simulink model "sampleModel1439"  (R2023a)
settings: Solver=VariableStepAuto  StartTime=0.0  StopTime=10.0  RelTol=1e-3
libraries: hdlsllib x4, simulink x1
settings Model: Creator=user1  LastModifiedBy=user1

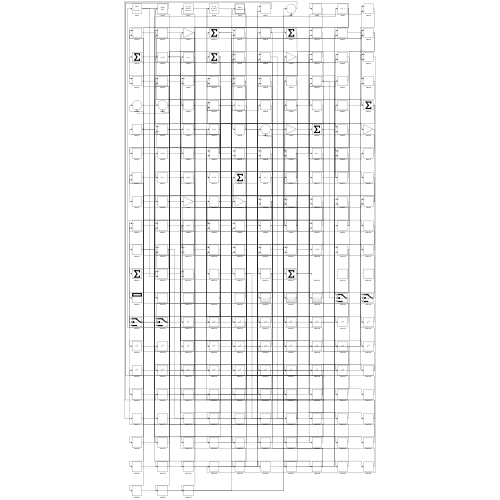
[thumbnail: Simulink's stored preview of the top-level diagram]
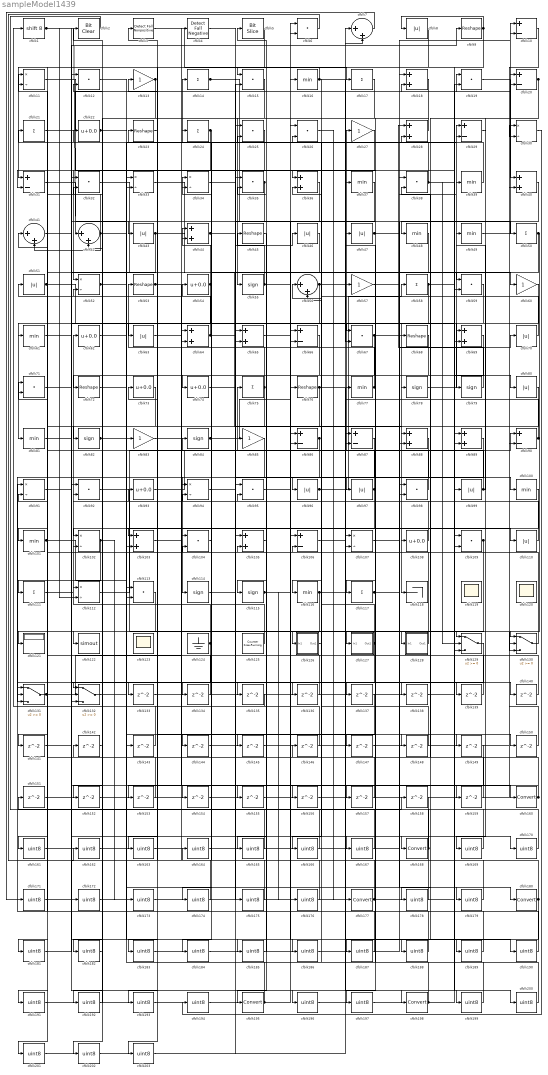
== system sampleModel1439 ==
  cfblk1 : ArithShift  BitShiftNumber=8
  cfblk{10,20,29,31,66,86..87,90,106} (9 alike) : Sum  Inputs=+-
  cfblk{16,37,39,48..49,61,77,81,100..101,116} (11 alike) : MinMax
  cfblk{11,30,33..34,52,91,94,102,107,112} (10 alike) : Product  Inputs=*/  RndMeth=Zero  SaturateOnIntegerOverflow=on
  cfblk{18,28,36,40,44,64..65,69,88..89,103,105} (12 alike) : Sum
  cfblk{6,12,15,19,25..26,32,35,38,59,67,71,92,95,98,104,109,113} (18 alike) : DotProduct  OutDataTypeStr=Inherit: Inherit via internal rule
  cfblk{22,54,62,73..74,93,108} (7 alike) : Bias  Bias=0.0  SaturateOnIntegerOverflow=off
  cfblk{8,43,46..47,51,63,70,80,96..97,99,110} (12 alike) : Abs  SaturateOnIntegerOverflow=off
  cfblk{14,17,21,24,50,58,75,111,117} (9 alike) : Sum  Inputs=+
  cfblk{55,78..79,82,84,114..115} (7 alike) : Signum
  cfblk118 : Terminator
  cfblk119 : Scope
      settings: Floating=on
  cfblk120 : Scope
      settings: Floating=on
  cfblk121 : Display
  cfblk122 : ToWorkspace  VariableName=simout  SaveFormat=Timeseries  SampleTime=-1
  cfblk123 : Scope
      settings: Floating=on
  cfblk124 : Ground
  cfblk125 : hdlsllib/Sources/Counter Free-Running  NumBits=16  tsamp=-1
  cfblk126 : Subsystem
      settings: LibrarySourceBlock=|
      | hdlsllib/Ports &
      | Subsystems/Subsystem
  cfblk127 : Subsystem
      settings: LibrarySourceBlock=|
      | hdlsllib/Ports &
      | Subsystems/Subsystem
  cfblk128 : Subsystem
      settings: LibrarySourceBlock=|
      | hdlsllib/Ports &
      | Subsystems/Subsystem
  cfblk{129..132} (4 alike) : Switch  SaturateOnIntegerOverflow=off  InputSameDT=off
  cfblk{13,27,57,60,83,85} (6 alike) : Gain
  cfblk{133..159} (27 alike) : Delay  SampleTime=1
  cfblk{160,168,177,180,195,198} (6 alike) : DataTypeConversion  SaturateOnIntegerOverflow=off  RndMeth=Floor
  cfblk{161..167,169..176,178..179,181..194,196..197,199..203} (38 alike) : DataTypeConversion  OutDataTypeStr=uint8  SaturateOnIntegerOverflow=off  RndMeth=Floor
  cfblk2 : simulink/Logic and Bit Operations/Bit Clear  iBit=0
      settings: LibrarySourceBlock=|
      | hdlsllib/Logic and Bit
      | Operations/Bit Clear
  cfblk{9,23,45,53,68,72,76} (7 alike) : Reshape
  cfblk3 : hdlsllib/Logic and Bit Operations/Detect Fall Nonpositive  vinit=0  OutDataTypeStr=boolean
  cfblk4 : hdlsllib/Logic and Bit Operations/Detect Fall Negative  vinit=0  OutDataTypeStr=boolean
  cfblk{7,41..42,56} (4 alike) : Sum  Inputs=|++
  cfblk5 : hdlsllib/Logic and Bit Operations/Bit Slice  lidx=7  ridx=0
  wires:
  cfblk17/1 -> cfblk55/1
  cfblk40/1 -> cfblk48/1
  cfblk86/1 -> cfblk114/1, cfblk131/3
  cfblk54/1 -> cfblk81/1, cfblk44/2
  cfblk79/1 -> cfblk28/1
  cfblk28/1 -> cfblk36/1
  cfblk32/1 -> cfblk118/1
  cfblk24/1 -> cfblk52/1, cfblk184/1
  cfblk1/1 -> cfblk42/1, cfblk59/1, cfblk112/2
  cfblk49/1 -> cfblk10/1
  cfblk124/1 -> cfblk62/1, cfblk203/1
  cfblk75/1 -> cfblk53/1, cfblk101/1
  cfblk35/1 -> cfblk132/3, cfblk144/1
  cfblk52/1 -> cfblk33/2, cfblk157/1
  cfblk97/1 -> cfblk3/1, cfblk41/1, cfblk156/1
  cfblk31/1 -> cfblk83/1
  cfblk50/1 -> cfblk130/1, cfblk135/1
  cfblk55/1 -> cfblk45/1, cfblk69/2, cfblk130/3
  cfblk89/1 -> cfblk195/1
  cfblk51/1 -> cfblk108/1, cfblk185/1
  cfblk96/1 -> cfblk58/1, cfblk166/1
  cfblk5/1 -> cfblk31/1
  cfblk69/1 -> cfblk78/1
  cfblk58/1 -> cfblk61/1, cfblk150/1
  cfblk90/1 -> cfblk27/1, cfblk82/1
  cfblk116/1 -> cfblk149/1, cfblk161/1
  cfblk42/1 -> cfblk11/1, cfblk41/2, cfblk29/2
  cfblk38/1 -> cfblk14/1, cfblk80/1, cfblk129/2
  cfblk3/1 -> cfblk17/1
  cfblk98/1 -> cfblk37/1
  cfblk78/1 -> cfblk29/1
  cfblk110/1 -> cfblk2/1
  cfblk14/1 -> cfblk68/1, cfblk167/1
  cfblk43/1 -> cfblk121/1, cfblk67/2
  cfblk113/1 -> cfblk122/1
  cfblk44/1 -> cfblk88/1, cfblk107/2
  cfblk125/1 -> cfblk84/1
  cfblk101/1 -> cfblk143/1, cfblk170/1
  cfblk70/1 -> cfblk21/1
  cfblk93/1 -> cfblk75/1
  cfblk27/1 -> cfblk31/2
  cfblk128/1(Out1) -> cfblk73/1
  cfblk41/1 -> cfblk67/1
  cfblk47/1 -> cfblk97/1, cfblk10/2
  cfblk112/1 -> cfblk64/1
  cfblk15/1 -> cfblk72/1
  cfblk77/1 -> cfblk54/1, cfblk34/1
  cfblk59/1 -> cfblk116/1
  cfblk16/1 -> cfblk15/1, cfblk60/1, cfblk126/1(In1)
  cfblk115/1 -> cfblk19/1, cfblk176/1
  cfblk111/1 -> cfblk112/1
  cfblk23/1 -> cfblk63/1
  cfblk107/1 -> cfblk39/1
  cfblk102/1 -> cfblk111/1, cfblk173/1
  cfblk22/1 -> cfblk59/2, cfblk148/1
  cfblk19/1 -> cfblk40/1
  cfblk11/1 -> cfblk109/1
  cfblk56/1 -> cfblk28/2, cfblk133/1
  cfblk33/1 -> cfblk76/1
  cfblk72/1 -> cfblk110/1
  cfblk127/1(Out1) -> cfblk56/1, cfblk131/2
  cfblk60/1 -> cfblk79/1
  cfblk106/1 -> cfblk198/1
  cfblk18/1 -> cfblk117/1
  cfblk48/1 -> cfblk94/1
  cfblk109/1 -> cfblk129/1, cfblk163/1
  cfblk92/1 -> cfblk127/1(In1)
  cfblk53/1 -> cfblk139/1, cfblk140/1
  cfblk76/1 -> cfblk115/1, cfblk128/1(In1)
  cfblk57/1 -> cfblk160/1
  cfblk130/1 -> cfblk71/1
  cfblk103/1 -> cfblk90/1
  cfblk108/1 -> cfblk24/1
  cfblk84/1 -> cfblk16/1, cfblk34/2
  cfblk94/1 -> cfblk18/2
  cfblk67/1 -> cfblk74/1, cfblk20/2, cfblk103/2
  cfblk36/1 -> cfblk86/2
  cfblk82/1 -> cfblk132/1, cfblk147/1
  cfblk21/1 -> cfblk20/1
  cfblk71/1 -> cfblk9/1
  cfblk39/1 -> cfblk5/1
  cfblk95/1 -> cfblk168/1
  cfblk117/1 -> cfblk70/1, cfblk179/1
  cfblk20/1 -> cfblk69/1, cfblk188/1
  cfblk37/1 -> cfblk102/1
  cfblk13/1 -> cfblk113/2, cfblk202/1
  cfblk26/1 -> cfblk177/1
  cfblk10/1 -> cfblk30/2
  cfblk114/1 -> cfblk46/1
  cfblk64/1 -> cfblk51/1, cfblk88/2, cfblk13/1
  cfblk74/1 -> cfblk100/1
  cfblk131/1 -> cfblk4/1, cfblk154/1
  cfblk4/1 -> cfblk50/1
  cfblk9/1 -> cfblk43/1, cfblk103/1, cfblk8/1, cfblk129/3
  cfblk12/1 -> cfblk180/1
  cfblk99/1 -> cfblk49/1, cfblk44/1
  cfblk126/1(Out1) -> cfblk56/2
  cfblk68/1 -> cfblk96/1
  cfblk133/1 -> cfblk109/2
  cfblk46/1 -> cfblk134/1
  cfblk134/1 -> cfblk33/1
  cfblk135/1 -> cfblk1/1
  cfblk81/1 -> cfblk136/1
  cfblk136/1 -> cfblk92/1
  cfblk88/1 -> cfblk137/1
  cfblk83/1 -> cfblk138/1
  cfblk139/1 -> cfblk18/1
  cfblk140/1 -> cfblk11/2
  cfblk85/1 -> cfblk141/1
  cfblk142/1 -> cfblk52/2
  cfblk143/1 -> cfblk102/2
  cfblk144/1 -> cfblk86/1
  cfblk132/1 -> cfblk145/1
  cfblk145/1 -> cfblk30/1
  cfblk146/1 -> cfblk131/1
  cfblk147/1 -> cfblk90/2
  cfblk148/1 -> cfblk36/2
  cfblk150/1 -> cfblk130/2
  cfblk151/1 -> cfblk98/1
  cfblk80/1 -> cfblk152/1
  cfblk152/1 -> cfblk64/2
  cfblk153/1 -> cfblk71/2
  cfblk154/1 -> cfblk94/2
  cfblk45/1 -> cfblk155/1
  cfblk155/1 -> cfblk40/2
  cfblk156/1 -> cfblk19/2
  cfblk157/1 -> cfblk42/2
  cfblk2/1 -> cfblk158/1
  cfblk63/1 -> cfblk159/1
  cfblk159/1 -> cfblk23/1
  cfblk160/1 -> cfblk153/1, cfblk38/2
  cfblk161/1 -> cfblk57/1
  cfblk6/1 -> cfblk162/1
  cfblk162/1 -> cfblk98/2
  cfblk163/1 -> cfblk6/1
  cfblk158/1 -> cfblk164/1
  cfblk164/1 -> cfblk6/2
  cfblk105/1 -> cfblk165/1
  cfblk165/1 -> cfblk151/1
  cfblk166/1 -> cfblk105/1
  cfblk167/1 -> cfblk105/2
  cfblk168/1 -> cfblk142/1, cfblk85/1
  cfblk29/1 -> cfblk169/1
  cfblk169/1 -> cfblk95/1
  cfblk170/1 -> cfblk95/2
  cfblk7/1 -> cfblk171/1
  cfblk171/1 -> cfblk32/1
  cfblk61/1 -> cfblk172/1
  cfblk172/1 -> cfblk7/1
  cfblk173/1 -> cfblk7/2
  cfblk104/1 -> cfblk174/1
  cfblk174/1 -> cfblk93/1
  cfblk34/1 -> cfblk175/1
  cfblk175/1 -> cfblk104/1
  cfblk176/1 -> cfblk104/2
  cfblk177/1 -> cfblk35/2, cfblk47/1, cfblk32/2, cfblk99/1
  cfblk149/1 -> cfblk178/1
  cfblk178/1 -> cfblk26/1
  cfblk179/1 -> cfblk26/2
  cfblk180/1 -> cfblk132/2, cfblk107/1, cfblk197/1
  cfblk73/1 -> cfblk181/1
  cfblk181/1 -> cfblk12/1
  cfblk100/1 -> cfblk182/1
  cfblk182/1 -> cfblk12/2
  cfblk25/1 -> cfblk183/1
  cfblk183/1 -> cfblk38/1
  cfblk184/1 -> cfblk25/1
  cfblk185/1 -> cfblk25/2
  cfblk91/1 -> cfblk186/1
  cfblk186/1 -> cfblk146/1
  cfblk129/1 -> cfblk187/1
  cfblk187/1 -> cfblk91/1
  cfblk188/1 -> cfblk91/2
  cfblk65/1 -> cfblk189/1
  cfblk189/1 -> cfblk22/1
  cfblk62/1 -> cfblk190/1
  cfblk190/1 -> cfblk65/1
  cfblk8/1 -> cfblk191/1
  cfblk191/1 -> cfblk65/2
  cfblk66/1 -> cfblk192/1
  cfblk192/1 -> cfblk92/2
  cfblk137/1 -> cfblk193/1
  cfblk193/1 -> cfblk66/1
  cfblk30/1 -> cfblk194/1
  cfblk194/1 -> cfblk66/2
  cfblk195/1 -> cfblk113/1, cfblk199/1
  cfblk141/1 -> cfblk196/1
  cfblk196/1 -> cfblk89/1
  cfblk197/1 -> cfblk89/2
  cfblk198/1 -> cfblk35/1, cfblk77/1
  cfblk199/1 -> cfblk106/1
  cfblk138/1 -> cfblk200/1
  cfblk200/1 -> cfblk106/2
  cfblk87/1 -> cfblk201/1
  cfblk201/1 -> cfblk15/2
  cfblk202/1 -> cfblk87/1
  cfblk203/1 -> cfblk87/2

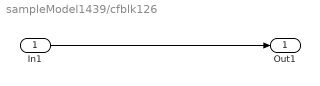
== system sampleModel1439/cfblk126 ==
  In1 : Inport
  Out1 : Outport
  wires:
  In1/1 -> Out1/1

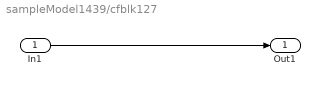
== system sampleModel1439/cfblk127 ==
  In1 : Inport
  Out1 : Outport
  wires:
  In1/1 -> Out1/1

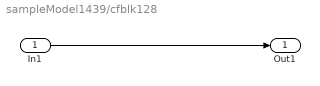
== system sampleModel1439/cfblk128 ==
  In1 : Inport
  Out1 : Outport
  wires:
  In1/1 -> Out1/1
